simulink model "Transversal"  (Simulink 7.1)
settings: Solver=ode45  StartTime=0.0  StopTime=120.0  RelTol=1e-4
settings Model: Creator=Meisel  LastModifiedBy=Meisel

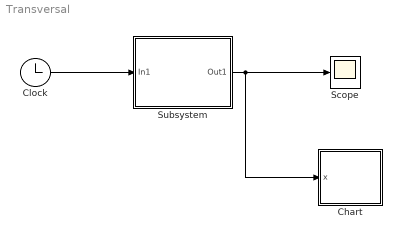
== system Transversal ==
  Chart : Stateflow chart
  Clock : Clock
  Scope : Scope
  Subsystem : Subsystem  mask{c=1000, l0=0.1, m=1.5}
  wires:
  Clock/1 -> Subsystem/1(In1)
  Subsystem/1(Out1) -> Scope/1, Chart/1(x)

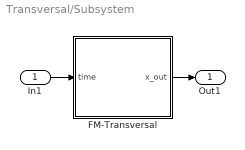
== system Transversal/Subsystem ==
  In1 : Inport
  FM-Transversal : Stateflow chart
  Out1 : Outport
  wires:
  In1/1 -> FM-Transversal/1(time)
  FM-Transversal/1(x_out) -> Out1/1

== stateflow chart Subsystem/FM-Transversal ==
  settings: updateMethod=CONTINUOUS
  state Swing
    during:
    // derivatives
    x_dot=v;
    v_dot=Acc();
    // output
    x_out=x;
  note: Die Size und Datentypparameter
      | von Rückgabeparametern
      | (z.B. a und f müssen im DataExplorer)
      | explizit gesetzt werden.
  (default) -> Swing : {InitCond();
      |  ml.xyFederMassePlot("init", k, l0);}
  Swing -> Swing : [time>=0.1 && StartCond()]
      | {Start();}
  data: a function_output double size=k,2; f function_output boolean; time input double; k constant double =50; c parameter double; l0 parameter double; m parameter double; x_out output double size=k,2; x local double size=k,2; v local double size=k,2
  data k settings: description=Anzahl der Massen
  data c settings: description=Federkonstante
  data l0 settings: description=Federlänge
  data m settings: description=Masse
  data x settings: updateMethod=SF_CONTINUOUS_TIME_DATA
  data v settings: updateMethod=SF_CONTINUOUS_TIME_DATA
  function a = Acc:
    | function a = Acc
    | 
    | a=zeros(k, 2);  %% Größe (size = k,2) im Data Explorer setzen !!!!
    | 
    | % Das erste und letzte Element sollen fix sein.
    | a(1,:)=[0,0];     % statt  a(1,1)=0;   a(1,2)=0; 
    | a(k,:)=[0,0];     % stat   a(k,1)=0;   a(k,2)=0;
    | 
    | for i=2:k-1
    |     a(i,:) = CalcAcceleration(i);
    | end
    | 
    | 
    | 
    | function ai = CalcAcceleration(i) 
    |     
    |     ai=[0,0];
    |     
    |     % Kraftvektor durch Vorgänger
    |     FVorg = -norm((x(i,:)-x(i-1,:))-l0) * (x(i,:)-x(i-1,:))/norm(x(i,:)-x(i-1,:));
    |     
    |     % Kraftvektor durch Vorgänger
    |     FNach = norm((x(i+1,:)-x(i,:))-l0) * (x(i+1,:)-x(i,:))/norm(x(i+1,:)-x(i,:));
    |     
    |     % Gesamtkraftvektor
    |     F=FVorg+FNach;
    |     
    |     % Beschleunigung
    |     ai=F/m;
  function InitCond:
    | function InitCond
    | 
    | for i=1:k
    |     x(i,1)= l0*(i-1);
    |     x(i,2)= 0;
    | end
  function Start:
    | function Start
    | 
    | x(1,2)=0.002*l0;
  function f=StartCond:
    | function f=StartCond
    | 
    | % F=boolean muss im Model Explorer explitit gesetzt werden
    | f = x(1,1)==0 && x(1,2)==0;

== stateflow chart Chart ==
  state Draw
    during:
    ml.xyFederMassePlot("update", x)
  (default) -> Draw
  data: x input double
